simulink model "PFC_69C_03_06_V01_3Phase_3_2KW"  (R2022b)
settings: Solver=FixedStepAuto  StartTime=0.0  StopTime=Inf  RelTol=1e-3  EnableMultiTasking=on
model workspace (MAT data in the model file):
  ADC_Gain = 1241.21212121
  DAC_Gain = 0.000805860805861
  Inductor_Current_Divider_Gain_Phase_A = 33.4
  Inductor_Current_Divider_Gain_Phase_B = 33.4
  Vbulk_Divider_Gain = 276.854928018
  Vin_Divider_Gain = 556.17352614
undefined symbols (not defined in the file or in its folder): GPTRIP1SEL, GPTRIP2SEL, SCI_A_Transmit, SCI_A_Transmit_Current_Suffix, SCI_A_Transmit_one_shot_Suffix, SCI_A_Transmit_Polarity_Suffix, SCI_A_Transmit_relay_Suffix, SCI_A_Transmit_Vbulk_Suffix, SCI_A_Transmit_Vin_rms_Suffix, SCI_A_Transmit_Vin_Suffix, SCI_A_Transmit_Vmid_Suffix, SCI_A_Transmit_Vp_Suffix, SCI_A_Transmit_Vpfc_Suffix, TZ1, TZ2
libraries: c280xlib x38, c2802xlib x34, simulink x17, c2000lib x1
(part 3 of 8)

== system PFC_69C_03_06_V01_3Phase_3_2KW/PWM Update @50KHz/Fixed Duty update_Phase_A ==
  note: if PWM is 0, have to set Soft Start flag to 1 so that we can have a softstart at the next start up.
  function : TriggerPort  TriggerType=function-call  VariantControl=(inherit)
  Archive : Subsystem  Commented=on
  Constant : Constant
  Constant1 : Constant  Value=50
  Constant2 : Constant  Value=10
  Data Store Read : DataStoreRead  DataStoreName=ePWM2A_CMPA_Phase_A  IndexOptions=Index vector (dialog)  Indices=1  OutputSizes=1
  Data Store Read1 : DataStoreRead  DataStoreName=PFC_en_Phase_A  IndexOptions=Index vector (dialog)  Indices=1  OutputSizes=1
  Data Store Read2 : DataStoreRead  DataStoreName=Relay_started  IndexOptions=Index vector (dialog)  Indices=1  OutputSizes=1
  Data Store Read4 : DataStoreRead  DataStoreName=One_Shot_Bar  IndexOptions=Index vector (dialog)  Indices=1  OutputSizes=1
  Data Store Write : DataStoreWrite  DataStoreName=debug  IndexOptions=Index vector (dialog)  Indices=1  OutputSizes=1
  Gain2 : Gain  Gain=0.5
  Product1 : Product  Inputs=5  OutDataTypeStr=double
  Subsystem1 : Subsystem
  ePWM1 : c2802xlib/ePWM  PwmType=C2000  useModule=ePWM2  ePWMxLINKTBPRD=Not Linked  periodUnits=Clock cycles  timerSource=Input port  timerPeriod_clk=1799  timerPeriod_sec=0.0001  tbshadow=Counter equals to zero  countingMode=Up  phaseActiveEnable=Disable  phaseDirection=Count down after sync  phaseActive=0  synchronizationEnable=off  dcaevt1Sync=off  dcbevt1Sync=off  synchronizationOption=Disable  dcbevt1SyncOut=off  dcaevt1SyncOut=off  cmpdSyncOut=off  cmpcSyncOut=off  cmpbSyncOut=off  zeroSyncOut=off  swfSyncOut=off  perSynchronizationOption=Counter equals to period (CTR=PRD)  clockPrescale=1  HSclockPrescale=1  enswap=off  ePWMxAStatus=on  ePWMxAactionLogic1=Set  ePWMxAactionLogic2=Do nothing  ePWMxAactionLogic3=Clear  ePWMxAactionLogic4=Set  ePWMxAactionLogic5=Do nothing  ePWMxAactionLogic6=Do nothing  ePWMxACSFenable=off  ePWMxACSFvalue=Forcing disable  ePWMxASFreload=Zero  ePWMxBStatus=off  ePWMxBactionLogic1=Set  ePWMxBactionLogic2=Clear  ePWMxBactionLogic3=Clear  ePWMxBactionLogic4=Do nothing  ePWMxBactionLogic5=Clear  ePWMxBactionLogic6=Set  ePWMxBCSFenable=off  ePWMxBCSFvalue=Forcing disable  ePWMxBSFreload=Zero  ePWNxBOutWay=off  ePWMxLINKCMPA=Not Linked  CMPAUnits=Clock cycles  CMPASource=Input port  CMPAValue_per=50  CMPAValue_clk=0  enCMPAshadow=Counter equals to zero (CTR=Zero)  ePWMxLINKCMPB=Not Linked  CMPBUnits=Clock cycles  CMPBSource=Input port  CMPBValue_per=50  CMPBValue_clk=0  enCMPBshadow=Counter equals to zero (CTR=Zero)  ePWMxLINKCMPC=Not Linked  CMPCUnits=Clock cycles  CMPCSource=Specify via dialog  CMPCValue_per=50  CMPCValue_clk=32000  enCMPCshadow=Counter equals to zero (CTR=Zero)  ePWMxLINKCMPD=Not Linked  CMPDUnits=Clock cycles  CMPDSource=Specify via dialog  CMPDValue_per=50  CMPDValue_clk=32000  enCMPDshadow=Counter equals to zero (CTR=Zero)  enableDBePWMxA=off  enableDBePWMxB=off  enhalfcycle=off  DBpolarity=Active high (AH)  DBedgeDelay=Positive  DBSource_ePWMxA=ePWMxA  DBSource_ePWMxB=ePWMxA  DBPeriodUnits=Clock cycles  DBperiodSource=Specify via dialog  REDperiod=0  FEDperiod=0  REDperiod_sec=0  FEDperiod_sec=0  LoadModeDBRED=Immediate without using shadow  LoadModeDBFED=Immediate without using shadow  adcstartModuleA=on  adcrequestEventA=First event  adcstartEventA=Counter is incrementing and equals to the compare B register (CTRU=CMPB)  adcstartEventA_type2=Digital Compare Module A Event 1 start of conversion (DCAEVT1.soc)  adcstartModuleB=off  adcrequestEventB=First event  adcstartEventB=Counter equals to zero (CTR=Zero)  adcstartEventB_type2=Counter equals to zero (CTR=Zero)  intEn=on  intPrd=First event  intSel=Counter equals to zero (CTR=Zero)  intSel_type2=Counter equals to zero (CTR=Zero)  hrpe=off  enHRPWM=off  HRPWM_LoadMode=Counter equals to period (CTR=PRD)  HRPWM_CTLMode=Duty or Period control mode  HRPWM_EDGMode=Both edge  hrpeb=off  enHRPWMB=off  HRPWM_LoadModeB=Counter equals to zero (CTR=ZERO)  HRPWM_CTLModeB=Duty or Period control mode  HRPWM_EDGModeB=Both edge  enHRDBRED=off  enHRDBFED=off  enSFO=on  enautoconv=on  chopperEnable=off  chopperFrequency=1  chopperFirstwidth=1  chopperDuty=12.5%  tripZonesource=Specify via dialog  tzselOSHT1=off  tzselOSHT2=off  tzselOSHT3=off  tzselOSHDCAEV1=off  tzselOSHDCBEV1=off  tzselCBC1=off  tzselCBC2=off  tzselCBC3=off  tzselCBCDCAEV2=off  tzselCBCDCBEV2=off  tzselOSHT4=off  tzselOSHT5=off  tzselOSHT6=off  tzselCBC4=off  tzselCBC5=off  tzselCBC6=off  enTzOstIntr=off  enTzCbcIntr=off  enTzDCAEVT1Intr=off  enTzDCAEVT2Intr=off  enTzDCBEVT1Intr=off  enTzDCBEVT2Intr=off  ePWMxAforced=No action  ePWMxBforced=No action  DCAEVT1forced=Low  DCBEVT1forced=No action  DCAEVT2forced=Low  DCBEVT2forced=No action  dcah=COMP1OUT input  dcal=COMP2OUT input  dcbh=Trip Zone 1 input (TZ1)  dcbl=Trip Zone 1 input (TZ1)  dcah_type2=GPTRIP1SEL/(TZ1)  dcal_type2=GPTRIP2SEL/(TZ2)  dcbh_type2=GPTRIP1SEL/(TZ1)  dcbl_type2=GPTRIP2SEL/(TZ2)  gendcaevt1=DCAL=high and DCAH=don't care  gendcaevt2=DCAH=high and DCAL=don't care  gendcbevt1=Event disabled  gendcbevt2=Event disabled  dcaevt1src=DCAEVT1 with sync  dcaevt2src=DCAEVT2 with async  dcbevt1src=DCBEVT1 with sync  dcbevt2src=DCBEVT2 with sync  pulsesel=Counter equals to zero (CTR=Zero)  blankinv=off  blankoffset=0  blankwidth=0  evsrcsel=Filtered version of DCAEVT1 (DCAEVT1FILT)  encape=off
      settings: LibrarySourceBlock=c2806xlib/ePWM
  wires:
  Data Store Read4/1 -> Product1/3
  Subsystem1/1(Out1) -> ePWM1/1
  Constant1/1 -> Subsystem1/1(Frequency(kHz))
  Gain2/1 -> ePWM1/3
  Product1/1 -> ePWM1/2, Gain2/1, Data Store Write/1
  Data Store Read/1 -> Product1/1
  Data Store Read1/1 -> Product1/2
  Data Store Read2/1 -> Product1/4
  Constant2/1 -> Subsystem1/2(Duty(%))
  Constant/1 -> Product1/5

== system PFC_69C_03_06_V01_3Phase_3_2KW/PWM Update @50KHz/Fixed Duty update_Phase_B_Test ==
  note: if PWM is 0, have to set Soft Start flag to 1 so that we can have a softstart at the next start up.
  function : TriggerPort  TriggerType=function-call  VariantControl=(inherit)
  Archive : Subsystem  Commented=on
  Constant : Constant
  Constant1 : Constant  Value=50
  Constant2 : Constant  Value=10
  Data Store Read : DataStoreRead  DataStoreName=ePWM1A_CMPA_Phase_B  IndexOptions=Index vector (dialog)  Indices=1  OutputSizes=1
  Data Store Read1 : DataStoreRead  DataStoreName=PFC_en_Phase_B  IndexOptions=Index vector (dialog)  Indices=1  OutputSizes=1
  Data Store Read2 : DataStoreRead  DataStoreName=Relay_started  IndexOptions=Index vector (dialog)  Indices=1  OutputSizes=1
  Data Store Read4 : DataStoreRead  DataStoreName=One_Shot_Bar  IndexOptions=Index vector (dialog)  Indices=1  OutputSizes=1
  Data Store Write : DataStoreWrite  DataStoreName=debug  IndexOptions=Index vector (dialog)  Indices=1  OutputSizes=1
  Gain2 : Gain  Gain=0.5
  Product1 : Product  Inputs=5  OutDataTypeStr=double
  Subsystem1 : Subsystem
  ePWM1 : c2802xlib/ePWM  PwmType=C2000  useModule=ePWM1  ePWMxLINKTBPRD=Not Linked  periodUnits=Clock cycles  timerSource=Input port  timerPeriod_clk=1799  timerPeriod_sec=0.0001  tbshadow=Counter equals to zero  countingMode=Up  phaseActiveEnable=Disable  phaseDirection=Count down after sync  phaseActive=18  synchronizationEnable=off  dcaevt1Sync=off  dcbevt1Sync=off  synchronizationOption=Disable  dcbevt1SyncOut=off  dcaevt1SyncOut=off  cmpdSyncOut=off  cmpcSyncOut=off  cmpbSyncOut=off  zeroSyncOut=off  swfSyncOut=off  perSynchronizationOption=Counter equals to period (CTR=PRD)  clockPrescale=1  HSclockPrescale=1  enswap=off  ePWMxAStatus=on  ePWMxAactionLogic1=Set  ePWMxAactionLogic2=Do nothing  ePWMxAactionLogic3=Clear  ePWMxAactionLogic4=Set  ePWMxAactionLogic5=Do nothing  ePWMxAactionLogic6=Do nothing  ePWMxACSFenable=off  ePWMxACSFvalue=Forcing disable  ePWMxASFreload=Zero  ePWMxBStatus=off  ePWMxBactionLogic1=Set  ePWMxBactionLogic2=Clear  ePWMxBactionLogic3=Clear  ePWMxBactionLogic4=Do nothing  ePWMxBactionLogic5=Clear  ePWMxBactionLogic6=Set  ePWMxBCSFenable=off  ePWMxBCSFvalue=Forcing disable  ePWMxBSFreload=Zero  ePWNxBOutWay=off  ePWMxLINKCMPA=Not Linked  CMPAUnits=Clock cycles  CMPASource=Input port  CMPAValue_per=50  CMPAValue_clk=0  enCMPAshadow=Counter equals to zero (CTR=Zero)  ePWMxLINKCMPB=Not Linked  CMPBUnits=Clock cycles  CMPBSource=Input port  CMPBValue_per=50  CMPBValue_clk=0  enCMPBshadow=Counter equals to zero (CTR=Zero)  ePWMxLINKCMPC=Not Linked  CMPCUnits=Clock cycles  CMPCSource=Specify via dialog  CMPCValue_per=50  CMPCValue_clk=32000  enCMPCshadow=Counter equals to zero (CTR=Zero)  ePWMxLINKCMPD=Not Linked  CMPDUnits=Clock cycles  CMPDSource=Specify via dialog  CMPDValue_per=50  CMPDValue_clk=32000  enCMPDshadow=Counter equals to zero (CTR=Zero)  enableDBePWMxA=off  enableDBePWMxB=off  enhalfcycle=off  DBpolarity=Active high (AH)  DBedgeDelay=Positive  DBSource_ePWMxA=ePWMxA  DBSource_ePWMxB=ePWMxA  DBPeriodUnits=Clock cycles  DBperiodSource=Specify via dialog  REDperiod=0  FEDperiod=0  REDperiod_sec=0  FEDperiod_sec=0  LoadModeDBRED=Immediate without using shadow  LoadModeDBFED=Immediate without using shadow  adcstartModuleA=off  adcrequestEventA=First event  adcstartEventA=Counter is incrementing and equals to the compare B register (CTRU=CMPB)  adcstartEventA_type2=Digital Compare Module A Event 1 start of conversion (DCAEVT1.soc)  adcstartModuleB=off  adcrequestEventB=First event  adcstartEventB=Counter equals to zero (CTR=Zero)  adcstartEventB_type2=Counter equals to zero (CTR=Zero)  intEn=off  intPrd=First event  intSel=Counter equals to zero (CTR=Zero)  intSel_type2=Counter equals to zero (CTR=Zero)  hrpe=off  enHRPWM=off  HRPWM_LoadMode=Counter equals to period (CTR=PRD)  HRPWM_CTLMode=Duty or Period control mode  HRPWM_EDGMode=Both edge  hrpeb=off  enHRPWMB=off  HRPWM_LoadModeB=Counter equals to zero (CTR=ZERO)  HRPWM_CTLModeB=Duty or Period control mode  HRPWM_EDGModeB=Both edge  enHRDBRED=off  enHRDBFED=off  enSFO=on  enautoconv=on  chopperEnable=off  chopperFrequency=1  chopperFirstwidth=1  chopperDuty=12.5%  tripZonesource=Specify via dialog  tzselOSHT1=off  tzselOSHT2=off  tzselOSHT3=off  tzselOSHDCAEV1=off  tzselOSHDCBEV1=off  tzselCBC1=off  tzselCBC2=off  tzselCBC3=off  tzselCBCDCAEV2=off  tzselCBCDCBEV2=off  tzselOSHT4=off  tzselOSHT5=off  tzselOSHT6=off  tzselCBC4=off  tzselCBC5=off  tzselCBC6=off  enTzOstIntr=off  enTzCbcIntr=off  enTzDCAEVT1Intr=off  enTzDCAEVT2Intr=off  enTzDCBEVT1Intr=off  enTzDCBEVT2Intr=off  ePWMxAforced=No action  ePWMxBforced=No action  DCAEVT1forced=No action  DCBEVT1forced=No action  DCAEVT2forced=Low  DCBEVT2forced=No action  dcah=COMP1OUT input  dcal=Trip Zone 2 input (TZ2)  dcbh=Trip Zone 1 input (TZ1)  dcbl=Trip Zone 1 input (TZ1)  dcah_type2=GPTRIP1SEL/(TZ1)  dcal_type2=GPTRIP2SEL/(TZ2)  dcbh_type2=GPTRIP1SEL/(TZ1)  dcbl_type2=GPTRIP2SEL/(TZ2)  gendcaevt1=Event disabled  gendcaevt2=DCAH=high and DCAL=don't care  gendcbevt1=Event disabled  gendcbevt2=Event disabled  dcaevt1src=DCAEVT1 with sync  dcaevt2src=DCAEVT2 with async  dcbevt1src=DCBEVT1 with sync  dcbevt2src=DCBEVT2 with sync  pulsesel=Counter equals to zero (CTR=Zero)  blankinv=off  blankoffset=0  blankwidth=0  evsrcsel=Filtered version of DCAEVT1 (DCAEVT1FILT)  encape=off
      settings: LibrarySourceBlock=c2806xlib/ePWM
  wires:
  Data Store Read4/1 -> Product1/3
  Subsystem1/1(Out1) -> ePWM1/1
  Constant1/1 -> Subsystem1/1(Frequency(kHz))
  Gain2/1 -> ePWM1/3
  Product1/1 -> ePWM1/2, Gain2/1, Data Store Write/1
  Data Store Read/1 -> Product1/1
  Data Store Read1/1 -> Product1/2
  Data Store Read2/1 -> Product1/4
  Constant2/1 -> Subsystem1/2(Duty(%))
  Constant/1 -> Product1/5

== system PFC_69C_03_06_V01_3Phase_3_2KW/PWM Update @50KHz/Fixed Duty update_Phase_C ==
  note: if PWM is 0, have to set Soft Start flag to 1 so that we can have a softstart at the next start up.
  function : TriggerPort  TriggerType=function-call  VariantControl=(inherit)
  Archive : Subsystem  Commented=on
  Constant : Constant
  Constant1 : Constant  Value=50
  Constant2 : Constant  Value=10
  Data Store Read : DataStoreRead  DataStoreName=ePWM3A_CMPA_Phase_C  IndexOptions=Index vector (dialog)  Indices=1  OutputSizes=1
  Data Store Read1 : DataStoreRead  DataStoreName=PFC_en_Phase_C  IndexOptions=Index vector (dialog)  Indices=1  OutputSizes=1
  Data Store Read2 : DataStoreRead  DataStoreName=Relay_started  IndexOptions=Index vector (dialog)  Indices=1  OutputSizes=1
  Data Store Read4 : DataStoreRead  DataStoreName=One_Shot_Bar  IndexOptions=Index vector (dialog)  Indices=1  OutputSizes=1
  Data Store Write : DataStoreWrite  DataStoreName=debug  IndexOptions=Index vector (dialog)  Indices=1  OutputSizes=1
  Gain2 : Gain  Gain=0.5
  Product1 : Product  Inputs=5  OutDataTypeStr=double
  Subsystem1 : Subsystem
  ePWM1 : c2802xlib/ePWM  PwmType=C2000  useModule=ePWM3  ePWMxLINKTBPRD=Not Linked  periodUnits=Clock cycles  timerSource=Input port  timerPeriod_clk=1799  timerPeriod_sec=0.0001  tbshadow=Counter equals to zero  countingMode=Up  phaseActiveEnable=Disable  phaseDirection=Count down after sync  phaseActive=36  synchronizationEnable=off  dcaevt1Sync=off  dcbevt1Sync=off  synchronizationOption=Disable  dcbevt1SyncOut=off  dcaevt1SyncOut=off  cmpdSyncOut=off  cmpcSyncOut=off  cmpbSyncOut=off  zeroSyncOut=off  swfSyncOut=off  perSynchronizationOption=Counter equals to period (CTR=PRD)  clockPrescale=1  HSclockPrescale=1  enswap=off  ePWMxAStatus=on  ePWMxAactionLogic1=Set  ePWMxAactionLogic2=Do nothing  ePWMxAactionLogic3=Clear  ePWMxAactionLogic4=Set  ePWMxAactionLogic5=Do nothing  ePWMxAactionLogic6=Do nothing  ePWMxACSFenable=off  ePWMxACSFvalue=Forcing disable  ePWMxASFreload=Zero  ePWMxBStatus=off  ePWMxBactionLogic1=Set  ePWMxBactionLogic2=Clear  ePWMxBactionLogic3=Clear  ePWMxBactionLogic4=Do nothing  ePWMxBactionLogic5=Clear  ePWMxBactionLogic6=Set  ePWMxBCSFenable=off  ePWMxBCSFvalue=Forcing disable  ePWMxBSFreload=Zero  ePWNxBOutWay=off  ePWMxLINKCMPA=Not Linked  CMPAUnits=Clock cycles  CMPASource=Input port  CMPAValue_per=50  CMPAValue_clk=0  enCMPAshadow=Counter equals to zero (CTR=Zero)  ePWMxLINKCMPB=Not Linked  CMPBUnits=Clock cycles  CMPBSource=Input port  CMPBValue_per=50  CMPBValue_clk=0  enCMPBshadow=Counter equals to zero (CTR=Zero)  ePWMxLINKCMPC=Not Linked  CMPCUnits=Clock cycles  CMPCSource=Specify via dialog  CMPCValue_per=50  CMPCValue_clk=32000  enCMPCshadow=Counter equals to zero (CTR=Zero)  ePWMxLINKCMPD=Not Linked  CMPDUnits=Clock cycles  CMPDSource=Specify via dialog  CMPDValue_per=50  CMPDValue_clk=32000  enCMPDshadow=Counter equals to zero (CTR=Zero)  enableDBePWMxA=off  enableDBePWMxB=off  enhalfcycle=off  DBpolarity=Active high (AH)  DBedgeDelay=Positive  DBSource_ePWMxA=ePWMxA  DBSource_ePWMxB=ePWMxA  DBPeriodUnits=Clock cycles  DBperiodSource=Specify via dialog  REDperiod=0  FEDperiod=0  REDperiod_sec=0  FEDperiod_sec=0  LoadModeDBRED=Immediate without using shadow  LoadModeDBFED=Immediate without using shadow  adcstartModuleA=off  adcrequestEventA=First event  adcstartEventA=Counter is incrementing and equals to the compare B register (CTRU=CMPB)  adcstartEventA_type2=Digital Compare Module A Event 1 start of conversion (DCAEVT1.soc)  adcstartModuleB=off  adcrequestEventB=First event  adcstartEventB=Counter equals to zero (CTR=Zero)  adcstartEventB_type2=Counter equals to zero (CTR=Zero)  intEn=off  intPrd=First event  intSel=Counter equals to zero (CTR=Zero)  intSel_type2=Counter equals to zero (CTR=Zero)  hrpe=off  enHRPWM=off  HRPWM_LoadMode=Counter equals to period (CTR=PRD)  HRPWM_CTLMode=Duty or Period control mode  HRPWM_EDGMode=Both edge  hrpeb=off  enHRPWMB=off  HRPWM_LoadModeB=Counter equals to zero (CTR=ZERO)  HRPWM_CTLModeB=Duty or Period control mode  HRPWM_EDGModeB=Both edge  enHRDBRED=off  enHRDBFED=off  enSFO=on  enautoconv=on  chopperEnable=off  chopperFrequency=1  chopperFirstwidth=1  chopperDuty=12.5%  tripZonesource=Specify via dialog  tzselOSHT1=off  tzselOSHT2=off  tzselOSHT3=off  tzselOSHDCAEV1=off  tzselOSHDCBEV1=off  tzselCBC1=off  tzselCBC2=off  tzselCBC3=off  tzselCBCDCAEV2=off  tzselCBCDCBEV2=off  tzselOSHT4=off  tzselOSHT5=off  tzselOSHT6=off  tzselCBC4=off  tzselCBC5=off  tzselCBC6=off  enTzOstIntr=off  enTzCbcIntr=off  enTzDCAEVT1Intr=off  enTzDCAEVT2Intr=off  enTzDCBEVT1Intr=off  enTzDCBEVT2Intr=off  ePWMxAforced=No action  ePWMxBforced=No action  DCAEVT1forced=No action  DCBEVT1forced=No action  DCAEVT2forced=No action  DCBEVT2forced=No action  dcah=Trip Zone 2 input (TZ2)  dcal=Trip Zone 2 input (TZ2)  dcbh=Trip Zone 1 input (TZ1)  dcbl=Trip Zone 1 input (TZ1)  dcah_type2=GPTRIP1SEL/(TZ1)  dcal_type2=GPTRIP2SEL/(TZ2)  dcbh_type2=GPTRIP1SEL/(TZ1)  dcbl_type2=GPTRIP2SEL/(TZ2)  gendcaevt1=Event disabled  gendcaevt2=Event disabled  gendcbevt1=Event disabled  gendcbevt2=Event disabled  dcaevt1src=DCAEVT1 with sync  dcaevt2src=DCAEVT2 with sync  dcbevt1src=DCBEVT1 with sync  dcbevt2src=DCBEVT2 with sync  pulsesel=Counter equals to zero (CTR=Zero)  blankinv=off  blankoffset=0  blankwidth=0  evsrcsel=Filtered version of DCAEVT1 (DCAEVT1FILT)  encape=off
      settings: LibrarySourceBlock=c2806xlib/ePWM
  wires:
  Subsystem1/1(Out1) -> ePWM1/1
  Constant1/1 -> Subsystem1/1(Frequency(kHz))
  Product1/1 -> ePWM1/2, Gain2/1, Data Store Write/1
  Data Store Read/1 -> Product1/1
  Data Store Read1/1 -> Product1/2
  Data Store Read4/1 -> Product1/3
  Data Store Read2/1 -> Product1/4
  Constant2/1 -> Subsystem1/2(Duty(%))
  Gain2/1 -> ePWM1/3
  Constant/1 -> Product1/5

== system PFC_69C_03_06_V01_3Phase_3_2KW/PWM Update @50KHz/Voltage loop PWM generation (Control) ==
  function : TriggerPort  TriggerType=function-call  VariantControl=(inherit)
  Data Store Read1 : DataStoreRead  DataStoreName=Relay_started  IndexOptions=Index vector (dialog)  Indices=1  OutputSizes=1
  Data Store Read7 : DataStoreRead  DataStoreName=PFC_en  IndexOptions=Index vector (dialog)  Indices=1  OutputSizes=1
  If : If  NumInputs=2  IfExpression=(u1==1) & (u2==1)  ShowElse=off
  If Action Subsystem : Subsystem  TreatAsAtomicUnit=on
  wires:
  Data Store Read7/1 -> If/1
  If/1 -> If Action Subsystem/Action
  Data Store Read1/1 -> If/2

== system PFC_69C_03_06_V01_3Phase_3_2KW/UART reporting @ 1Hz/Data_calculation ==
  function : TriggerPort  TriggerType=function-call  VariantControl=(inherit)
  DataCalculation_Phase_A : Subsystem  TreatAsAtomicUnit=on
  DataCalculation_Phase_B : Subsystem  TreatAsAtomicUnit=on
  DataCalculation_Phase_C : Subsystem  TreatAsAtomicUnit=on
  Function-Call Generator : simulink/Ports & Subsystems/Function-Call Generator  sample_time=-1  numberOfIterations=1  DisallowWideOutput=off
  Function-Call Split : FunctionCallSplit  IconShape=distinctive  NumOutputPorts=4  OutputPortLayout=default
  Vbulk&Vmid : Subsystem  TreatAsAtomicUnit=on
  wires:
  Function-Call Generator/1 -> Function-Call Split/1
  Function-Call Split/1 -> DataCalculation_Phase_A/Trigger
  Function-Call Split/2 -> DataCalculation_Phase_B/Trigger
  Function-Call Split/3 -> DataCalculation_Phase_C/Trigger
  Function-Call Split/4 -> Vbulk&Vmid/Trigger

== system PFC_69C_03_06_V01_3Phase_3_2KW/UART reporting @ 1Hz/Phase_A ==
  function : TriggerPort  TriggerType=function-call  VariantControl=(inherit)
  Duty_control_loop_Phase_A : Subsystem  TreatAsAtomicUnit=on
  Function-Call Generator : simulink/Ports & Subsystems/Function-Call Generator  sample_time=-1  numberOfIterations=1  DisallowWideOutput=off
  Function-Call Split : FunctionCallSplit  IconShape=distinctive  NumOutputPorts=6  OutputPortLayout=default
  Send Inductor_Current (A) : Subsystem  TreatAsAtomicUnit=on
  Send PFC_en_Phase_A : Subsystem  TreatAsAtomicUnit=on
  Send Vin (V) : Subsystem  Commented=on  TreatAsAtomicUnit=on
  Send Vin_rms (V) : Subsystem  TreatAsAtomicUnit=on
  Send control_loop_current : Subsystem  Commented=on  TreatAsAtomicUnit=on
  wires:
  Function-Call Generator/1 -> Function-Call Split/1
  Function-Call Split/1 -> Send Vin (V)/Trigger
  Function-Call Split/2 -> Send Inductor_Current (A)/Trigger
  Function-Call Split/3 -> Send Vin_rms (V)/Trigger
  Function-Call Split/4 -> Send control_loop_current/Trigger
  Function-Call Split/5 -> Send PFC_en_Phase_A/Trigger
  Function-Call Split/6 -> Duty_control_loop_Phase_A/Trigger

== system PFC_69C_03_06_V01_3Phase_3_2KW/UART reporting @ 1Hz/Phase_B ==
  function : TriggerPort  TriggerType=function-call  VariantControl=(inherit)
  Duty_control_loop_Phase_B : Subsystem  Commented=on  TreatAsAtomicUnit=on
  Function-Call Generator : simulink/Ports & Subsystems/Function-Call Generator  sample_time=-1  numberOfIterations=1  DisallowWideOutput=off
  Function-Call Split : FunctionCallSplit  IconShape=distinctive  NumOutputPorts=6  OutputPortLayout=default
  Send Inductor_Current (A) : Subsystem  TreatAsAtomicUnit=on
  Send PFC_en_Phase_B : Subsystem  Commented=on  TreatAsAtomicUnit=on
  Send Vin (V) : Subsystem  Commented=on  TreatAsAtomicUnit=on
  Send Vin_rms (V) : Subsystem  TreatAsAtomicUnit=on
  Send control loop current : Subsystem  Commented=on  TreatAsAtomicUnit=on
  wires:
  Function-Call Generator/1 -> Function-Call Split/1
  Function-Call Split/1 -> Send Vin (V)/Trigger
  Function-Call Split/2 -> Send Inductor_Current (A)/Trigger
  Function-Call Split/3 -> Send Vin_rms (V)/Trigger
  Function-Call Split/4 -> Send control loop current/Trigger
  Function-Call Split/5 -> Send PFC_en_Phase_B/Trigger
  Function-Call Split/6 -> Duty_control_loop_Phase_B/Trigger

== system PFC_69C_03_06_V01_3Phase_3_2KW/UART reporting @ 1Hz/Phase_C ==
  function : TriggerPort  TriggerType=function-call  VariantControl=(inherit)
  Duty_control_loop_Phase_C : Subsystem  Commented=on  TreatAsAtomicUnit=on
  Function-Call Generator : simulink/Ports & Subsystems/Function-Call Generator  sample_time=-1  numberOfIterations=1  DisallowWideOutput=off
  Function-Call Split : FunctionCallSplit  IconShape=distinctive  NumOutputPorts=6  OutputPortLayout=default
  Send Inductor_Current (A) : Subsystem  TreatAsAtomicUnit=on
  Send PFC_en_Phase_C : Subsystem  Commented=on  TreatAsAtomicUnit=on
  Send Vin (V) : Subsystem  Commented=on  TreatAsAtomicUnit=on
  Send Vin_rms (V) : Subsystem  TreatAsAtomicUnit=on
  Send control loop current : Subsystem  Commented=on  TreatAsAtomicUnit=on
  wires:
  Function-Call Generator/1 -> Function-Call Split/1
  Function-Call Split/1 -> Send Vin (V)/Trigger
  Function-Call Split/2 -> Send Inductor_Current (A)/Trigger
  Function-Call Split/3 -> Send Vin_rms (V)/Trigger
  Function-Call Split/4 -> Send control loop current/Trigger
  Function-Call Split/5 -> Send PFC_en_Phase_C/Trigger
  Function-Call Split/6 -> Duty_control_loop_Phase_C/Trigger

== system PFC_69C_03_06_V01_3Phase_3_2KW/UART reporting @ 1Hz/SCI_A_Transmit_function ==
  SCI_A_Transmit : TriggerPort  TriggerType=function-call  IsSimulinkFunction=on  FunctionName=SCI_A_Transmit  FunctionVisibility=scoped  VariantControl=(inherit)
  Add Constant{,1..4} (5 alike) : Bias  Bias=48  SaturateOnIntegerOverflow=off
  Constant : Constant  Value=10000
  MATLAB Function : MATLAB Function  TreatAsAtomicUnit=on
  Mux : Mux  Inputs=5
  SCI Transmit : c280xlib/SCI Transmit  sciModule=A  dataHead=''  dataTail=''  blockingMode=on  outputStatus=off
  u : ArgIn  DisableCoverage=on  ArgumentName=u
  wires:
  Mux/1 -> SCI Transmit/1
  Add Constant4/1 -> Mux/5
  Add Constant3/1 -> Mux/4
  Add Constant2/1 -> Mux/3
  Add Constant1/1 -> Mux/2
  Add Constant/1 -> Mux/1
  MATLAB Function/1(Digit_5) -> Add Constant/1
  MATLAB Function/2(Digit_4) -> Add Constant1/1
  MATLAB Function/3(Digit_3) -> Add Constant2/1
  MATLAB Function/4(Digit_2) -> Add Constant3/1
  MATLAB Function/5(Digit_1) -> Add Constant4/1
  Constant/1 -> MATLAB Function/2(Divider)
  u/1 -> MATLAB Function/1(Main_number)

== system PFC_69C_03_06_V01_3Phase_3_2KW/UART reporting @ 1Hz/SCI_A_Transmit_function1 ==
  note: 86 Decimal = 'V' in ASCII
  SCI_A_Transmit_Vbulk_Suffix : TriggerPort  TriggerType=function-call  IsSimulinkFunction=on  FunctionName=SCI_A_Transmit_Vbulk_Suffix  FunctionVisibility=scoped  VariantControl=(inherit)
  SCI Transmit : c280xlib/SCI Transmit  sciModule=A  dataHead=''  dataTail=10  blockingMode=on  outputStatus=off
  Vbulk : Constant  Value=[86 98 117 108 107]  OutDataTypeStr=uint8
  wires:
  Vbulk/1 -> SCI Transmit/1

== system PFC_69C_03_06_V01_3Phase_3_2KW/UART reporting @ 1Hz/SCI_A_Transmit_function10 ==
  SCI_A_Transmit_one_shot_Suffix : TriggerPort  TriggerType=function-call  IsSimulinkFunction=on  FunctionName=SCI_A_Transmit_relay_Suffix  FunctionVisibility=scoped  VariantControl=(inherit)
  P O L : Constant  Value=[82 69 76]  OutDataTypeStr=uint8
  SCI Transmit : c280xlib/SCI Transmit  sciModule=A  dataHead=''  dataTail=10  blockingMode=on  outputStatus=off
  wires:
  P O L/1 -> SCI Transmit/1

== system PFC_69C_03_06_V01_3Phase_3_2KW/UART reporting @ 1Hz/SCI_A_Transmit_function2 ==
  note: 65 Decimal = 'A' in ASCII
  SCI_A_Transmit_Current_Suffix : TriggerPort  TriggerType=function-call  IsSimulinkFunction=on  FunctionName=SCI_A_Transmit_Current_Suffix  FunctionVisibility=scoped  VariantControl=(inherit)
  Current : Constant  Value=[65]  OutDataTypeStr=uint8
  SCI Transmit : c280xlib/SCI Transmit  sciModule=A  dataHead=''  dataTail=10  blockingMode=on  outputStatus=off
  wires:
  Current/1 -> SCI Transmit/1

== system PFC_69C_03_06_V01_3Phase_3_2KW/UART reporting @ 1Hz/SCI_A_Transmit_function3 ==
  note: 86 Decimal = 'V' in ASCII
  SCI_A_Transmit_Vin_Suffix : TriggerPort  TriggerType=function-call  IsSimulinkFunction=on  FunctionName=SCI_A_Transmit_Vin_Suffix  FunctionVisibility=scoped  VariantControl=(inherit)
  SCI Transmit : c280xlib/SCI Transmit  sciModule=A  dataHead=''  dataTail=10  blockingMode=on  outputStatus=off
  Vin : Constant  Value=[86 105 110]  OutDataTypeStr=uint8
  wires:
  Vin/1 -> SCI Transmit/1

== system PFC_69C_03_06_V01_3Phase_3_2KW/UART reporting @ 1Hz/SCI_A_Transmit_function4 ==
  note: 86 Decimal = 'V' in ASCII
  SCI_A_Transmit_Vin_rms_Suffix : TriggerPort  TriggerType=function-call  IsSimulinkFunction=on  FunctionName=SCI_A_Transmit_Vin_rms_Suffix  FunctionVisibility=scoped  VariantControl=(inherit)
  SCI Transmit : c280xlib/SCI Transmit  sciModule=A  dataHead=''  dataTail=10  blockingMode=on  outputStatus=off
  Vrms : Constant  Value=[86 114 109 115]  OutDataTypeStr=uint8
  wires:
  Vrms/1 -> SCI Transmit/1

== system PFC_69C_03_06_V01_3Phase_3_2KW/UART reporting @ 1Hz/SCI_A_Transmit_function5 ==
  SCI_A_Transmit_Polarity_Suffix : TriggerPort  TriggerType=function-call  IsSimulinkFunction=on  FunctionName=SCI_A_Transmit_Polarity_Suffix  FunctionVisibility=scoped  VariantControl=(inherit)
  P O L : Constant  Value=[80 79 76]  OutDataTypeStr=uint8
  SCI Transmit : c280xlib/SCI Transmit  sciModule=A  dataHead=''  dataTail=10  blockingMode=on  outputStatus=off
  wires:
  P O L/1 -> SCI Transmit/1

== system PFC_69C_03_06_V01_3Phase_3_2KW/UART reporting @ 1Hz/SCI_A_Transmit_function6 ==
  SCI_A_Transmit_Vp_Suffix : TriggerPort  TriggerType=function-call  IsSimulinkFunction=on  FunctionName=SCI_A_Transmit_Vp_Suffix  FunctionVisibility=scoped  VariantControl=(inherit)
  SCI Transmit : c280xlib/SCI Transmit  sciModule=A  dataHead=''  dataTail=10  blockingMode=on  outputStatus=off
  "VP " : Constant  Value=[86 80]  OutDataTypeStr=uint8
  wires:
  "VP "/1 -> SCI Transmit/1

== system PFC_69C_03_06_V01_3Phase_3_2KW/UART reporting @ 1Hz/SCI_A_Transmit_function7 ==
  note: 86 Decimal = 'V' in ASCII
  SCI_A_Transmit_Vmid_Suffix : TriggerPort  TriggerType=function-call  IsSimulinkFunction=on  FunctionName=SCI_A_Transmit_Vmid_Suffix  FunctionVisibility=scoped  VariantControl=(inherit)
  SCI Transmit : c280xlib/SCI Transmit  sciModule=A  dataHead=''  dataTail=10  blockingMode=on  outputStatus=off
  Vmid : Constant  Value=[86 109 105 100]  OutDataTypeStr=uint8
  wires:
  Vmid/1 -> SCI Transmit/1

== system PFC_69C_03_06_V01_3Phase_3_2KW/UART reporting @ 1Hz/SCI_A_Transmit_function8 ==
  SCI_A_Transmit_Vpfc_Suffix : TriggerPort  TriggerType=function-call  IsSimulinkFunction=on  FunctionName=SCI_A_Transmit_Vpfc_Suffix  FunctionVisibility=scoped  VariantControl=(inherit)
  SCI Transmit : c280xlib/SCI Transmit  sciModule=A  dataHead=''  dataTail=10  blockingMode=on  outputStatus=off
  "VPFC " : Constant  Value=[86 80 70 67]  OutDataTypeStr=uint8
  wires:
  "VPFC "/1 -> SCI Transmit/1

== system PFC_69C_03_06_V01_3Phase_3_2KW/UART reporting @ 1Hz/SCI_A_Transmit_function9 ==
  SCI_A_Transmit_one_shot_Suffix : TriggerPort  TriggerType=function-call  IsSimulinkFunction=on  FunctionName=SCI_A_Transmit_one_shot_Suffix  FunctionVisibility=scoped  VariantControl=(inherit)
  P O L : Constant  Value=[79 78 69]  OutDataTypeStr=uint8
  SCI Transmit : c280xlib/SCI Transmit  sciModule=A  dataHead=''  dataTail=10  blockingMode=on  outputStatus=off
  wires:
  P O L/1 -> SCI Transmit/1

== system PFC_69C_03_06_V01_3Phase_3_2KW/UART reporting @ 1Hz/Send PFC_en ==
  function : TriggerPort  TriggerType=function-call  VariantControl=(inherit)
  Data Store Read : DataStoreRead  DataStoreName=PFC_en  IndexOptions=Index vector (dialog)  Indices=1  OutputSizes=1
  Function Caller1 : FunctionCaller  FunctionPrototype=SCI_A_Transmit(u)  InputArgumentSpecifications=<Enter example>  OutputArgumentSpecifications=<Enter example>
  Function Caller2 : FunctionCaller  FunctionPrototype=SCI_A_Transmit_Vpfc_Suffix()  InputArgumentSpecifications=<Enter example>  OutputArgumentSpecifications=<Enter example>
  wires:
  Data Store Read/1 -> Function Caller1/1

== system PFC_69C_03_06_V01_3Phase_3_2KW/UART reporting @ 1Hz/Send Relay_started ==
  function : TriggerPort  TriggerType=function-call  VariantControl=(inherit)
  Data Store Read : DataStoreRead  DataStoreName=Relay_started  IndexOptions=Index vector (dialog)  Indices=1  OutputSizes=1
  Function Caller1 : FunctionCaller  FunctionPrototype=SCI_A_Transmit(u)  InputArgumentSpecifications=<Enter example>  OutputArgumentSpecifications=<Enter example>
  Function Caller2 : FunctionCaller  FunctionPrototype=SCI_A_Transmit_relay_Suffix()  InputArgumentSpecifications=<Enter example>  OutputArgumentSpecifications=<Enter example>
  wires:
  Data Store Read/1 -> Function Caller1/1

== system PFC_69C_03_06_V01_3Phase_3_2KW/UART reporting @ 1Hz/Send Vbulk (V) ==
  function : TriggerPort  TriggerType=function-call  VariantControl=(inherit)
  Data Store Read : DataStoreRead  DataStoreName=Vbulk  IndexOptions=Index vector (dialog)  Indices=1  OutputSizes=1
  Function Caller1 : FunctionCaller  FunctionPrototype=SCI_A_Transmit(u)  InputArgumentSpecifications=<Enter example>  OutputArgumentSpecifications=<Enter example>
  Function Caller2 : FunctionCaller  FunctionPrototype=SCI_A_Transmit_Vbulk_Suffix()  InputArgumentSpecifications=<Enter example>  OutputArgumentSpecifications=<Enter example>
  wires:
  Data Store Read/1 -> Function Caller1/1

== system PFC_69C_03_06_V01_3Phase_3_2KW/UART reporting @ 1Hz/Send Vmid ==
  function : TriggerPort  TriggerType=function-call  VariantControl=(inherit)
  Data Store Read : DataStoreRead  DataStoreName=Vmid_Topside  IndexOptions=Index vector (dialog)  Indices=1  OutputSizes=1
  Function Caller1 : FunctionCaller  FunctionPrototype=SCI_A_Transmit(u)  InputArgumentSpecifications=<Enter example>  OutputArgumentSpecifications=<Enter example>
  Function Caller2 : FunctionCaller  FunctionPrototype=SCI_A_Transmit_Vmid_Suffix()  InputArgumentSpecifications=<Enter example>  OutputArgumentSpecifications=<Enter example>
  wires:
  Data Store Read/1 -> Function Caller1/1

== system PFC_69C_03_06_V01_3Phase_3_2KW/UART reporting @ 1Hz/Send one_shot_bar ==
  function : TriggerPort  TriggerType=function-call  VariantControl=(inherit)
  Data Store Read : DataStoreRead  DataStoreName=One_Shot_Bar  IndexOptions=Index vector (dialog)  Indices=1  OutputSizes=1
  Function Caller1 : FunctionCaller  FunctionPrototype=SCI_A_Transmit(u)  InputArgumentSpecifications=<Enter example>  OutputArgumentSpecifications=<Enter example>
  Function Caller2 : FunctionCaller  FunctionPrototype=SCI_A_Transmit_one_shot_Suffix()  InputArgumentSpecifications=<Enter example>  OutputArgumentSpecifications=<Enter example>
  wires:
  Data Store Read/1 -> Function Caller1/1

== system PFC_69C_03_06_V01_3Phase_3_2KW/Calibration,RMS, Fault Protection @5kHz/Calibration/Calibration_3phase ==
  function : TriggerPort  TriggerType=function-call  VariantControl=(inherit)
  Chart : Stateflow chart  TreatAsAtomicUnit=on
  Constant1 : Constant  Commented=on
  Data Store Read1 : DataStoreRead  DataStoreName=Calibration_Done_Phase_A  IndexOptions=Index vector (dialog)  Indices=1  OutputSizes=1
  Data Store Read2 : DataStoreRead  DataStoreName=Calibration_Done_Phase_B  IndexOptions=Index vector (dialog)  Indices=1  OutputSizes=1
  Data Store Read4 : DataStoreRead  DataStoreName=Calibration_Done_Phase_C  IndexOptions=Index vector (dialog)  Indices=1  OutputSizes=1
  Data Store Write : DataStoreWrite  DataStoreName=Calibration_Done  IndexOptions=Index vector (dialog)  Indices=1  OutputSizes=1
  wires:
  Chart/1(Calibration_Done) -> Data Store Write/1
  Data Store Read2/1 -> Chart/2(Calibration_Done_Phase_B)
  Data Store Read1/1 -> Chart/1(Calibration_Done_Phase_A)
  Data Store Read4/1 -> Chart/3(Calibration_Done_Phase_C)

== system PFC_69C_03_06_V01_3Phase_3_2KW/Calibration,RMS, Fault Protection @5kHz/Calibration/Calibration_Phase_A ==
  function : TriggerPort  TriggerType=function-call  VariantControl=(inherit)
  Chart1 : Stateflow chart  TreatAsAtomicUnit=on
  Constant1 : Constant  Value=10000
  Data Store Read4 : DataStoreRead  DataStoreName=Inductor_Current_ADC_Phase_A  IndexOptions=Index vector (dialog)  Indices=1  OutputSizes=1
  Data Store Read5 : DataStoreRead  DataStoreName=Calibration_Done_Phase_A  IndexOptions=Index vector (dialog)  Indices=1  OutputSizes=1
  Data Store Read6 : DataStoreRead  DataStoreName=Vin_ADC_Phase_A  IndexOptions=Index vector (dialog)  Indices=1  OutputSizes=1
  Data Store Write4 : DataStoreWrite  DataStoreName=Calibration_Done_Phase_A  IndexOptions=Index vector (dialog)  Indices=1  OutputSizes=1
  Data Store Write5 : DataStoreWrite  DataStoreName=Inductor_Current_1_65_ADC_Phase_A  IndexOptions=Index vector (dialog)  Indices=1  OutputSizes=1
  Data Store Write6 : DataStoreWrite  DataStoreName=Vin_1_65_ADC_Phase_A  IndexOptions=Index vector (dialog)  Indices=1  OutputSizes=1
  wires:
  Chart1/1(output_signal_1) -> Data Store Write5/1
  Chart1/2(output_signal_2) -> Data Store Write6/1
  Constant1/1 -> Chart1/4(Counter_for_calibration)
  Data Store Read5/1 -> Chart1/1("Calibration_Done ")
  Chart1/3(Calibration_Done) -> Data Store Write4/1
  Data Store Read6/1 -> Chart1/3(input_signal_2)
  Data Store Read4/1 -> Chart1/2(input_signal_1)

== system PFC_69C_03_06_V01_3Phase_3_2KW/Calibration,RMS, Fault Protection @5kHz/Calibration/Calibration_Phase_B ==
  function : TriggerPort  TriggerType=function-call  VariantControl=(inherit)
  Chart1 : Stateflow chart  TreatAsAtomicUnit=on
  Constant1 : Constant  Value=10000
  Data Store Read4 : DataStoreRead  DataStoreName=Inductor_Current_ADC_Phase_B  IndexOptions=Index vector (dialog)  Indices=1  OutputSizes=1
  Data Store Read5 : DataStoreRead  DataStoreName=Calibration_Done_Phase_B  IndexOptions=Index vector (dialog)  Indices=1  OutputSizes=1
  Data Store Read6 : DataStoreRead  DataStoreName=Vin_ADC_Phase_B  IndexOptions=Index vector (dialog)  Indices=1  OutputSizes=1
  Data Store Write4 : DataStoreWrite  DataStoreName=Calibration_Done_Phase_B  IndexOptions=Index vector (dialog)  Indices=1  OutputSizes=1
  Data Store Write5 : DataStoreWrite  DataStoreName=Inductor_Current_1_65_ADC_Phase_B  IndexOptions=Index vector (dialog)  Indices=1  OutputSizes=1
  Data Store Write6 : DataStoreWrite  DataStoreName=Vin_1_65_ADC_Phase_B  IndexOptions=Index vector (dialog)  Indices=1  OutputSizes=1
  wires:
  Chart1/1(output_signal_1) -> Data Store Write5/1
  Chart1/2(output_signal_2) -> Data Store Write6/1
  Constant1/1 -> Chart1/4(Counter_for_calibration)
  Data Store Read5/1 -> Chart1/1("Calibration_Done ")
  Chart1/3(Calibration_Done) -> Data Store Write4/1
  Data Store Read6/1 -> Chart1/3(input_signal_2)
  Data Store Read4/1 -> Chart1/2(input_signal_1)

== system PFC_69C_03_06_V01_3Phase_3_2KW/Calibration,RMS, Fault Protection @5kHz/Calibration/Calibration_Phase_C ==
  function : TriggerPort  TriggerType=function-call  VariantControl=(inherit)
  Chart1 : Stateflow chart  TreatAsAtomicUnit=on
  Constant1 : Constant  Value=10000
  Data Store Read4 : DataStoreRead  DataStoreName=Inductor_Current_ADC_Phase_C  IndexOptions=Index vector (dialog)  Indices=1  OutputSizes=1
  Data Store Read5 : DataStoreRead  DataStoreName=Calibration_Done_Phase_C  IndexOptions=Index vector (dialog)  Indices=1  OutputSizes=1
  Data Store Read6 : DataStoreRead  DataStoreName=Vin_ADC_Phase_C  IndexOptions=Index vector (dialog)  Indices=1  OutputSizes=1
  Data Store Write4 : DataStoreWrite  DataStoreName=Calibration_Done_Phase_C  IndexOptions=Index vector (dialog)  Indices=1  OutputSizes=1
  Data Store Write5 : DataStoreWrite  DataStoreName=Inductor_Current_1_65_ADC_Phase_C  IndexOptions=Index vector (dialog)  Indices=1  OutputSizes=1
  Data Store Write6 : DataStoreWrite  DataStoreName=Vin_1_65_ADC_Phase_C  IndexOptions=Index vector (dialog)  Indices=1  OutputSizes=1
  wires:
  Chart1/1(output_signal_1) -> Data Store Write5/1
  Chart1/2(output_signal_2) -> Data Store Write6/1
  Constant1/1 -> Chart1/4(Counter_for_calibration)
  Data Store Read5/1 -> Chart1/1("Calibration_Done ")
  Chart1/3(Calibration_Done) -> Data Store Write4/1
  Data Store Read6/1 -> Chart1/3(input_signal_2)
  Data Store Read4/1 -> Chart1/2(input_signal_1)

== system PFC_69C_03_06_V01_3Phase_3_2KW/Calibration,RMS, Fault Protection @5kHz/Fault checking/If Action Subsystem ==
  note: Input UVP: Input<50 V, Recovery > 46 V
      | Input OVP: Input > 200 V, Recovery < 196 V
      | Output Vbulk OVP: 1.2 * Vbulk_setpoint
      | Midpoint Vbulk OVP: 0.6 * Vbulk_setpoint
      | Input current OCP: Current > 30 A, Recovery < 29 A
  note: O/P Bulk_UVP-> working but still not perfect.
      | Add more conditons during start up(Not to trigger)
  Action Port : ActionPort  ActionPortLabel=if(u1 ==1)
  Bulk_OVP_Latch : Subsystem  TreatAsAtomicUnit=on
  Fault Check (Bulk UVP) : Subsystem  Commented=on  TreatAsAtomicUnit=on
  Function-Call Generator : simulink/Ports & Subsystems/Function-Call Generator  sample_time=-1  numberOfIterations=1  DisallowWideOutput=off
  Function-Call Split : FunctionCallSplit  IconShape=distinctive  NumOutputPorts=11  OutputPortLayout=default
  Mid(Bottom side)_OVP_Latc : Subsystem  TreatAsAtomicUnit=on
  Mid(Top side)_OVP_Latch : Subsystem  TreatAsAtomicUnit=on
  PFC_en_update_3Phase : Subsystem  TreatAsAtomicUnit=on
  PFC_en_update_Phase_A : Subsystem  TreatAsAtomicUnit=on
  PFC_en_update_Phase_B : Subsystem  TreatAsAtomicUnit=on
  PFC_en_update_Phase_C : Subsystem  TreatAsAtomicUnit=on
  Phase_A_Fault : Subsystem  TreatAsAtomicUnit=on
  Phase_B_Fault : Subsystem  TreatAsAtomicUnit=on
  Phase_C_Fault : Subsystem  TreatAsAtomicUnit=on
  wires:
  Function-Call Generator/1 -> Function-Call Split/1
  Function-Call Split/1 -> Fault Check (Bulk UVP)/Trigger
  Function-Call Split/2 -> Bulk_OVP_Latch/Trigger
  Function-Call Split/3 -> Mid(Top side)_OVP_Latch/Trigger
  Function-Call Split/4 -> Mid(Bottom side)_OVP_Latc/Trigger
  Function-Call Split/5 -> Phase_A_Fault/Trigger
  Function-Call Split/6 -> Phase_B_Fault/Trigger
  Function-Call Split/7 -> Phase_C_Fault/Trigger
  Function-Call Split/8 -> PFC_en_update_Phase_A/Trigger
  Function-Call Split/9 -> PFC_en_update_Phase_B/Trigger
  Function-Call Split/10 -> PFC_en_update_Phase_C/Trigger
  Function-Call Split/11 -> PFC_en_update_3Phase/Trigger

== system PFC_69C_03_06_V01_3Phase_3_2KW/Calibration,RMS, Fault Protection @5kHz/Polarity & Near Zero check/Polarity_Near_zero_Phase_A ==
  note: Unit in Volt
  function : TriggerPort  TriggerType=function-call  VariantControl=(inherit)
  Chart : Stateflow chart  TreatAsAtomicUnit=on
  Constant7 : Constant  Value=0
  Data Store Read2 : DataStoreRead  DataStoreName=Vin_ADC_Average_Phase_A  IndexOptions=Index vector (dialog)  Indices=1  OutputSizes=1
  Data Store Read5 : DataStoreRead  DataStoreName=Vin_1_65_ADC_Phase_A  IndexOptions=Index vector (dialog)  Indices=1  OutputSizes=1
  Data Store Write1 : DataStoreWrite  DataStoreName=Near_Zero_Bar_Phase_A  IndexOptions=Index vector (dialog)  Indices=1  OutputSizes=1
  Data Store Write3 : DataStoreWrite  DataStoreName=Polarity_Phase_A  IndexOptions=Index vector (dialog)  Indices=1  OutputSizes=1
  Near Zero_7V_Analog : Constant  Value=7
  Near_zero : c280xlib/Digital Output  Commented=on  GPIO_Number=GPIO24~GPIO31  GPIO_Bit0=off  GPIO_BIT0_Toggle=off  GPIO_Bit1=on  GPIO_BIT1_Toggle=off  GPIO_Bit2=off  GPIO_BIT2_Toggle=off  GPIO_Bit3=off  GPIO_BIT3_Toggle=off  GPIO_Bit4=off  GPIO_BIT4_Toggle=off  GPIO_Bit5=off  GPIO_BIT5_Toggle=off  GPIO_Bit6=off  GPIO_BIT6_Toggle=off  GPIO_Bit7=off  GPIO_BIT7_Toggle=off
  Polarity : c280xlib/Digital Output  GPIO_Number=GPIO24~GPIO31  GPIO_Bit0=off  GPIO_BIT0_Toggle=off  GPIO_Bit1=on  GPIO_BIT1_Toggle=off  GPIO_Bit2=off  GPIO_BIT2_Toggle=off  GPIO_Bit3=off  GPIO_BIT3_Toggle=off  GPIO_Bit4=off  GPIO_BIT4_Toggle=off  GPIO_Bit5=off  GPIO_BIT5_Toggle=off  GPIO_Bit6=off  GPIO_BIT6_Toggle=off  GPIO_Bit7=off  GPIO_BIT7_Toggle=off
  Subtract2 : Sum  Inputs=+-
  Volt to Number : Subsystem
  wires:
  Constant7/1 -> Chart/2(Vref)
  Volt to Number/1(Out1) -> Chart/3(VZCD_Gap)
  Chart/2(Near_zero) -> Data Store Write1/1
  Near Zero_7V_Analog/1 -> Volt to Number/1(In1)
  Chart/1(Polarity) -> Polarity/1, Data Store Write3/1
  Data Store Read5/1 -> Subtract2/2
  Data Store Read2/1 -> Subtract2/1
  Subtract2/1 -> Chart/1(input)

== system PFC_69C_03_06_V01_3Phase_3_2KW/Calibration,RMS, Fault Protection @5kHz/Polarity & Near Zero check/Polarity_Near_zero_Phase_B ==
  note: Unit in Volt
  function : TriggerPort  TriggerType=function-call  VariantControl=(inherit)
  Chart : Stateflow chart  TreatAsAtomicUnit=on
  Constant7 : Constant  Value=0
  Data Store Read2 : DataStoreRead  DataStoreName=Vin_ADC_Average_Phase_B  IndexOptions=Index vector (dialog)  Indices=1  OutputSizes=1
  Data Store Read5 : DataStoreRead  DataStoreName=Vin_1_65_ADC_Phase_B  IndexOptions=Index vector (dialog)  Indices=1  OutputSizes=1
  Data Store Write1 : DataStoreWrite  DataStoreName=Near_Zero_Bar_Phase_B  IndexOptions=Index vector (dialog)  Indices=1  OutputSizes=1
  Data Store Write3 : DataStoreWrite  DataStoreName=Polarity_Phase_B  IndexOptions=Index vector (dialog)  Indices=1  OutputSizes=1
  Near Zero_7V_Analog : Constant  Value=7
  Near_zero : c280xlib/Digital Output  Commented=on  GPIO_Number=GPIO16~GPIO23  GPIO_Bit0=off  GPIO_BIT0_Toggle=off  GPIO_Bit1=off  GPIO_BIT1_Toggle=off  GPIO_Bit2=off  GPIO_BIT2_Toggle=off  GPIO_Bit3=off  GPIO_BIT3_Toggle=off  GPIO_Bit4=off  GPIO_BIT4_Toggle=off  GPIO_Bit5=off  GPIO_BIT5_Toggle=off  GPIO_Bit6=on  GPIO_BIT6_Toggle=off  GPIO_Bit7=off  GPIO_BIT7_Toggle=off
  Polarity : c280xlib/Digital Output  Commented=on  GPIO_Number=GPIO24~GPIO31  GPIO_Bit0=off  GPIO_BIT0_Toggle=off  GPIO_Bit1=on  GPIO_BIT1_Toggle=off  GPIO_Bit2=off  GPIO_BIT2_Toggle=off  GPIO_Bit3=off  GPIO_BIT3_Toggle=off  GPIO_Bit4=off  GPIO_BIT4_Toggle=off  GPIO_Bit5=off  GPIO_BIT5_Toggle=off  GPIO_Bit6=off  GPIO_BIT6_Toggle=off  GPIO_Bit7=off  GPIO_BIT7_Toggle=off
  Subtract2 : Sum  Inputs=+-
  Volt to Number : Subsystem
  wires:
  Constant7/1 -> Chart/2(Vref)
  Volt to Number/1(Out1) -> Chart/3(VZCD_Gap)
  Chart/2(Near_zero) -> Near_zero/1, Data Store Write1/1
  Near Zero_7V_Analog/1 -> Volt to Number/1(In1)
  Chart/1(Polarity) -> Polarity/1, Data Store Write3/1
  Data Store Read5/1 -> Subtract2/2
  Data Store Read2/1 -> Subtract2/1
  Subtract2/1 -> Chart/1(input)

== system PFC_69C_03_06_V01_3Phase_3_2KW/Calibration,RMS, Fault Protection @5kHz/Polarity & Near Zero check/Polarity_Near_zero_Phase_C ==
  note: Unit in Volt
  function : TriggerPort  TriggerType=function-call  VariantControl=(inherit)
  Chart : Stateflow chart  TreatAsAtomicUnit=on
  Constant7 : Constant  Value=0
  Data Store Read2 : DataStoreRead  DataStoreName=Vin_ADC_Average_Phase_C  IndexOptions=Index vector (dialog)  Indices=1  OutputSizes=1
  Data Store Read5 : DataStoreRead  DataStoreName=Vin_1_65_ADC_Phase_C  IndexOptions=Index vector (dialog)  Indices=1  OutputSizes=1
  Data Store Write1 : DataStoreWrite  DataStoreName=Near_Zero_Bar_Phase_C  IndexOptions=Index vector (dialog)  Indices=1  OutputSizes=1
  Data Store Write3 : DataStoreWrite  DataStoreName=Polarity_Phase_C  IndexOptions=Index vector (dialog)  Indices=1  OutputSizes=1
  Near Zero_7V_Analog : Constant  Value=7
  Near_zero : c280xlib/Digital Output  Commented=on  GPIO_Number=GPIO16~GPIO23  GPIO_Bit0=off  GPIO_BIT0_Toggle=off  GPIO_Bit1=off  GPIO_BIT1_Toggle=off  GPIO_Bit2=off  GPIO_BIT2_Toggle=off  GPIO_Bit3=off  GPIO_BIT3_Toggle=off  GPIO_Bit4=off  GPIO_BIT4_Toggle=off  GPIO_Bit5=off  GPIO_BIT5_Toggle=off  GPIO_Bit6=on  GPIO_BIT6_Toggle=off  GPIO_Bit7=off  GPIO_BIT7_Toggle=off
  Polarity : c280xlib/Digital Output  Commented=on  GPIO_Number=GPIO24~GPIO31  GPIO_Bit0=off  GPIO_BIT0_Toggle=off  GPIO_Bit1=on  GPIO_BIT1_Toggle=off  GPIO_Bit2=off  GPIO_BIT2_Toggle=off  GPIO_Bit3=off  GPIO_BIT3_Toggle=off  GPIO_Bit4=off  GPIO_BIT4_Toggle=off  GPIO_Bit5=off  GPIO_BIT5_Toggle=off  GPIO_Bit6=off  GPIO_BIT6_Toggle=off  GPIO_Bit7=off  GPIO_BIT7_Toggle=off
  Subtract2 : Sum  Inputs=+-
  Volt to Number : Subsystem
  wires:
  Constant7/1 -> Chart/2(Vref)
  Volt to Number/1(Out1) -> Chart/3(VZCD_Gap)
  Chart/2(Near_zero) -> Near_zero/1, Data Store Write1/1
  Near Zero_7V_Analog/1 -> Volt to Number/1(In1)
  Chart/1(Polarity) -> Polarity/1, Data Store Write3/1
  Data Store Read5/1 -> Subtract2/2
  Data Store Read2/1 -> Subtract2/1
  Subtract2/1 -> Chart/1(input)

== system PFC_69C_03_06_V01_3Phase_3_2KW/Calibration,RMS, Fault Protection @5kHz/Relay control/ADC Gain ==
  In1 : Inport
  Gain : Gain  Gain=ADC_Gain
  Gain1 : Gain  Gain=1/Vin_Divider_Gain
  Out1 : Outport
  wires:
  Gain1/1 -> Gain/1
  In1/1 -> Gain1/1
  Gain/1 -> Out1/1
